simulink model "amplificatorul"  (R2023b)
settings: Solver=VariableStepAuto  StartTime=0.0  StopTime=10.0  RelTol=1e-3
settings Model: Creator=diana.forrai  LastModifiedBy=diana.forrai

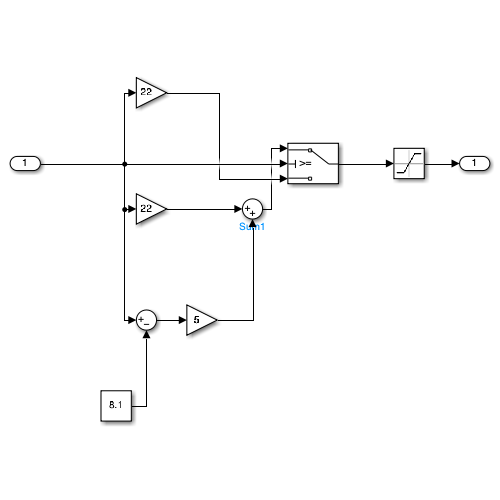
[thumbnail: Simulink's stored preview of the top-level diagram]
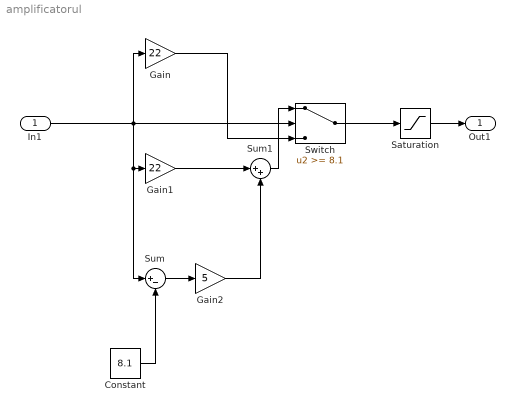
== system amplificatorul ==
  In1 : Inport
  Constant : Constant  Value=8.1
  Gain : Gain  Gain=22
  Gain1 : Gain  Gain=22
  Gain2 : Gain  Gain=5
  Saturation : Saturate  UpperLimit=22  LowerLimit=0
  Sum : Sum  Inputs=|+-
  Sum1 : Sum  Inputs=|++
  Switch : Switch  Threshold=8.1  SaturateOnIntegerOverflow=off  InputSameDT=off
  Out1 : Outport
  wires:
  Sum/1 -> Gain2/1
  Constant/1 -> Sum/2
  Gain2/1 -> Sum1/2
  Gain1/1 -> Sum1/1
  Switch/1 -> Saturation/1
  Saturation/1 -> Out1/1
  Sum1/1 -> Switch/1
  In1/1 -> Sum/1, Gain1/1, Gain/1, Switch/2
  Gain/1 -> Switch/3
